simulink model "automata_learning_boiler"  (R2021b)
settings: Solver=VariableStepAuto  StartTime=0.0  StopTime=10.0  RelTol=1e-3
settings Model: Creator=Falk  LastModifiedBy=Falk

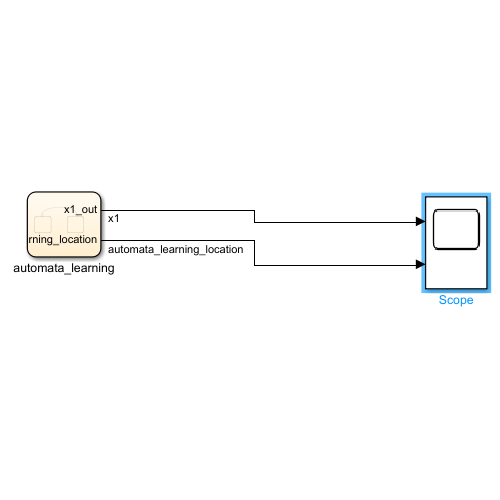
[thumbnail: Simulink's stored preview of the top-level diagram]
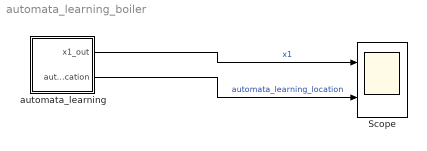
== system automata_learning_boiler ==
  Scope : Scope  NumInputPorts=2
  automata_learning : Stateflow chart  TreatAsAtomicUnit=on
  wires:
  automata_learning/1(x1_out) -> Scope/1  "x1"
  automata_learning/2(automata_learning_location) -> Scope/2  "automata_learning_location"

== stateflow chart automata_learning_boiler/automata_learning ==
  settings: updateMethod=CONTINUOUS
  state loc1
    du:
    x1_dot = 0.4988 * x1 + 0.4988;
    x1_out=x1;
    automata_learning_location =1;
  state loc2
    du:
    x1_dot = 0.000000000000255 - 0.5013 * x1;
    x1_out=x1;
    automata_learning_location =2;
  loc1 -> loc2 : [-0.03989 * x1 + 1.0 < 0.0]
  (default) -> loc1 : {x1 = 0.0;}
  loc2 -> loc1 : [-0.05013 * x1 + 1.0 > 0.0]
  data: x1_out output; x1 local; automata_learning_location output
  data x1 settings: updateMethod=SF_CONTINUOUS_TIME_DATA
